simulink model "alc"  (R2019b)
settings: Solver=FixedStepDiscrete  StartTime=0.0  StopTime=Tsim  FixedStep=0.02  RelTol=1e-3
InitFcn:
  | addpath('C:\tsdct\ETAS\ASCET\V6_1_4\target\psl\simulink_block')
libraries: psl_proxy_lib x1
settings Model: Creator=IGG2BP  LastModifiedBy=IGG2BP

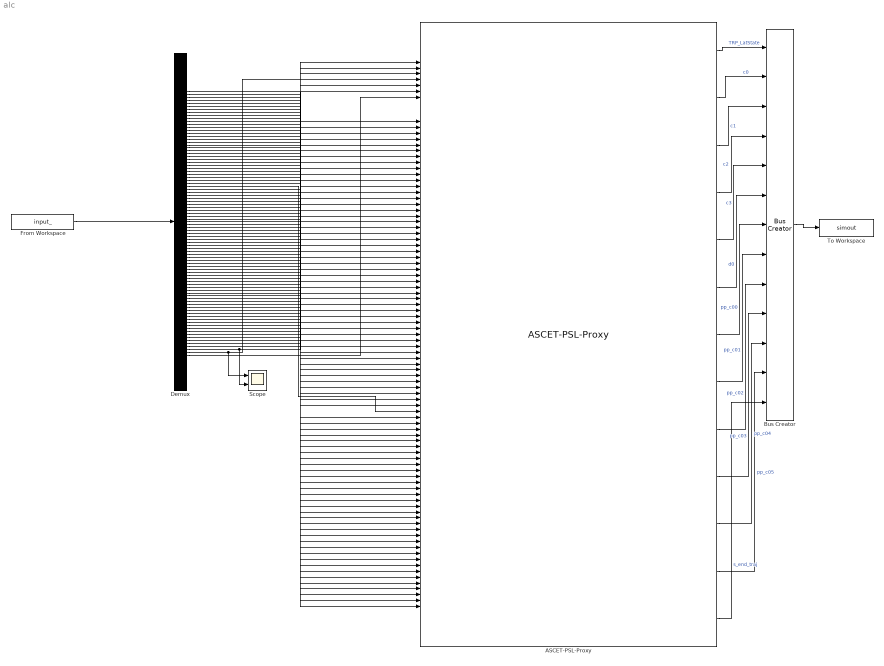
== system alc ==
  ASCET-PSL-Proxy : psl_proxy_lib/ASCET-PSL-Proxy  Description=ASCET-PSL Proxy S-Function Block  dll_name=LSMLat_PSL_Sim.ascet_psl  dcm_files=parameters.dcm|  datalog_file=datalog.mdf  log_level=info  csvDataLog=off  ignoreWrongVersion=off  measureAll=on
      settings: SourceProductName=ASCET-PSL
  Bus Creator : BusCreator  Inputs=13
  Demux : Demux  Outputs=91
  From Workspace : FromWorkspace  VariableName=input_  OutDataTypeStr=double
  Scope : Scope  NumInputPorts=2
  To Workspace : ToWorkspace  VariableName=simout  SaveFormat=Timeseries  SampleTime=-1
  wires:
  Demux/2 -> ASCET-PSL-Proxy/14
  Demux/3 -> ASCET-PSL-Proxy/36
  Demux/4 -> ASCET-PSL-Proxy/38
  Demux/5 -> ASCET-PSL-Proxy/40
  Demux/6 -> ASCET-PSL-Proxy/42
  Demux/7 -> ASCET-PSL-Proxy/44
  Demux/8 -> ASCET-PSL-Proxy/46
  Demux/9 -> ASCET-PSL-Proxy/48
  Demux/10 -> ASCET-PSL-Proxy/50
  Demux/11 -> ASCET-PSL-Proxy/52
  Demux/18 -> ASCET-PSL-Proxy/28
  Demux/12 -> ASCET-PSL-Proxy/16
  Demux/13 -> ASCET-PSL-Proxy/18
  Demux/14 -> ASCET-PSL-Proxy/20
  Demux/15 -> ASCET-PSL-Proxy/22
  Demux/16 -> ASCET-PSL-Proxy/24
  Demux/17 -> ASCET-PSL-Proxy/26
  Demux/19 -> ASCET-PSL-Proxy/30
  Demux/20 -> ASCET-PSL-Proxy/32
  Demux/21 -> ASCET-PSL-Proxy/34
  Demux/22 -> ASCET-PSL-Proxy/54
  Demux/23 -> ASCET-PSL-Proxy/76
  Demux/24 -> ASCET-PSL-Proxy/78
  Demux/25 -> ASCET-PSL-Proxy/80
  Demux/26 -> ASCET-PSL-Proxy/82
  Demux/27 -> ASCET-PSL-Proxy/84
  Demux/28 -> ASCET-PSL-Proxy/86
  Demux/29 -> ASCET-PSL-Proxy/88
  Demux/30 -> ASCET-PSL-Proxy/90
  Demux/31 -> ASCET-PSL-Proxy/92
  Demux/32 -> ASCET-PSL-Proxy/56
  Demux/33 -> ASCET-PSL-Proxy/58
  Demux/34 -> ASCET-PSL-Proxy/60
  Demux/35 -> ASCET-PSL-Proxy/62
  Demux/36 -> ASCET-PSL-Proxy/64
  Demux/37 -> ASCET-PSL-Proxy/66
  Demux/38 -> ASCET-PSL-Proxy/68
  Demux/39 -> ASCET-PSL-Proxy/70
  Demux/40 -> ASCET-PSL-Proxy/72
  Demux/41 -> ASCET-PSL-Proxy/74
  Demux/42 -> ASCET-PSL-Proxy/15
  Demux/43 -> ASCET-PSL-Proxy/37
  Demux/44 -> ASCET-PSL-Proxy/39
  Demux/45 -> ASCET-PSL-Proxy/41
  Demux/46 -> ASCET-PSL-Proxy/43
  Demux/47 -> ASCET-PSL-Proxy/45
  Demux/48 -> ASCET-PSL-Proxy/47
  Demux/49 -> ASCET-PSL-Proxy/49
  Demux/50 -> ASCET-PSL-Proxy/51
  Demux/51 -> ASCET-PSL-Proxy/53
  Demux/52 -> ASCET-PSL-Proxy/17
  Demux/53 -> ASCET-PSL-Proxy/19
  Demux/54 -> ASCET-PSL-Proxy/21
  Demux/55 -> ASCET-PSL-Proxy/23
  Demux/56 -> ASCET-PSL-Proxy/25
  Demux/57 -> ASCET-PSL-Proxy/27
  Demux/58 -> ASCET-PSL-Proxy/29
  Demux/59 -> ASCET-PSL-Proxy/31
  Demux/60 -> ASCET-PSL-Proxy/33
  Demux/61 -> ASCET-PSL-Proxy/35
  Demux/62 -> ASCET-PSL-Proxy/55
  Demux/63 -> ASCET-PSL-Proxy/77
  Demux/64 -> ASCET-PSL-Proxy/79
  Demux/65 -> ASCET-PSL-Proxy/81
  Demux/66 -> ASCET-PSL-Proxy/83
  Demux/67 -> ASCET-PSL-Proxy/85
  Demux/68 -> ASCET-PSL-Proxy/87
  Demux/69 -> ASCET-PSL-Proxy/89
  Demux/70 -> ASCET-PSL-Proxy/91
  Demux/71 -> ASCET-PSL-Proxy/93
  Demux/72 -> ASCET-PSL-Proxy/57
  Demux/73 -> ASCET-PSL-Proxy/59
  Demux/74 -> ASCET-PSL-Proxy/61
  Demux/75 -> ASCET-PSL-Proxy/63
  Demux/76 -> ASCET-PSL-Proxy/65
  Demux/77 -> ASCET-PSL-Proxy/67
  Demux/78 -> ASCET-PSL-Proxy/69
  Demux/79 -> ASCET-PSL-Proxy/71
  Demux/80 -> ASCET-PSL-Proxy/73
  Demux/81 -> ASCET-PSL-Proxy/75
  Demux/83 -> ASCET-PSL-Proxy/12
  Demux/84 -> ASCET-PSL-Proxy/13
  Demux/85 -> ASCET-PSL-Proxy/6
  Demux/86 -> ASCET-PSL-Proxy/2
  Demux/87 -> ASCET-PSL-Proxy/1
  Demux/88 -> ASCET-PSL-Proxy/3
  From Workspace/1 -> Demux/1
  Demux/82 -> ASCET-PSL-Proxy/11
  Bus Creator/1 -> To Workspace/1
  ASCET-PSL-Proxy/1 -> Bus Creator/1  "TRP_LatState"
  ASCET-PSL-Proxy/2 -> Bus Creator/2  "c0"
  ASCET-PSL-Proxy/3 -> Bus Creator/3  "c1"
  ASCET-PSL-Proxy/4 -> Bus Creator/4  "c2"
  ASCET-PSL-Proxy/5 -> Bus Creator/5  "c3"
  ASCET-PSL-Proxy/6 -> Bus Creator/6  "d0"
  ASCET-PSL-Proxy/7 -> Bus Creator/7  "pp_c00"
  ASCET-PSL-Proxy/8 -> Bus Creator/8  "pp_c01"
  ASCET-PSL-Proxy/9 -> Bus Creator/9  "pp_c02"
  ASCET-PSL-Proxy/10 -> Bus Creator/10  "pp_c03"
  ASCET-PSL-Proxy/11 -> Bus Creator/11  "pp_c04"
  ASCET-PSL-Proxy/12 -> Bus Creator/12  "pp_c05"
  ASCET-PSL-Proxy/13 -> Bus Creator/13  "s_end_traj"
  Demux/89 -> Scope/2, ASCET-PSL-Proxy/5
  Demux/90 -> Scope/1, ASCET-PSL-Proxy/4
  Demux/91 -> ASCET-PSL-Proxy/7
